simulink model "SmartTraffic"  (R2024b)
settings: Solver=VariableStepAuto  StartTime=0.0  StopTime=10.0  RelTol=1e-3
values from neighbouring files (symbols this model uses):
  dt = 1    [initTraffic.m]
  L_road = 5    [initTraffic.m]
  serviceRate = 2    [genTrafficData.m]    (also in initTraffic.m = 1)
libraries: fuzblock x1
settings Model: Creator=AJCaps  LastModifiedBy=AJCaps

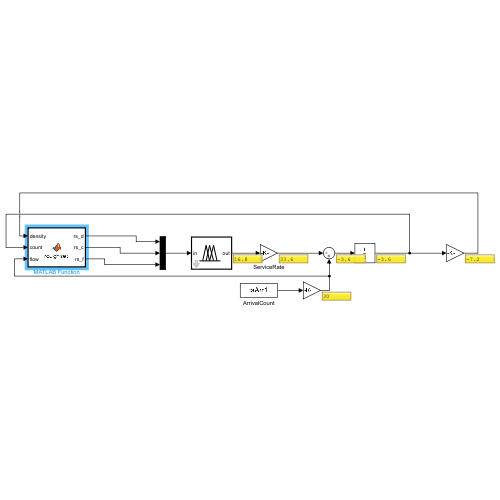
[thumbnail: Simulink's stored preview of the top-level diagram]
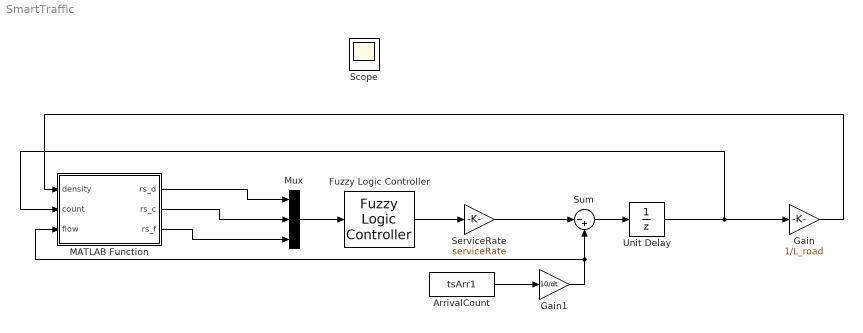
== system SmartTraffic ==
  ArrivalCount : FromWorkspace  VariableName=tsArr1
  Fuzzy Logic Controller : fuzblock/Fuzzy Logic  Controller  FIS='traffic_controller'  OutputSampleNumber=101  DataType=double  FuzzifiedInputs=off  RuleFiringStrengths=off  RuleOutputs=off  AggregatedOutputs=off  SimulateUsing=Interpreted execution  OutOfRangeInputValueMessage=warning  NoRuleFiredMessage=warning  EmptyOutputFuzzySetMessage=warning
  Gain : Gain  Gain=1/L_road
  Gain1 : Gain  Gain=10/dt
  MATLAB Function : MATLAB Function  TreatAsAtomicUnit=on
  Mux : Mux  Inputs=3
  ServiceRate : Gain  Gain=serviceRate
  Sum : Sum  Inputs=|-+
  Unit Delay : UnitDelay  SampleTime=-1  HasFrameUpgradeWarning=on
  Scope : Scope
  wires:
  Gain/1 -> MATLAB Function/1(density)
  Gain1/1 -> Sum/2, MATLAB Function/3(flow)
  MATLAB Function/1(rs_d) -> Mux/1
  Mux/1 -> Fuzzy Logic Controller/1
  Fuzzy Logic Controller/1 -> ServiceRate/1
  ArrivalCount/1 -> Gain1/1
  ServiceRate/1 -> Sum/1
  Sum/1 -> Unit Delay/1
  Unit Delay/1 -> MATLAB Function/2(count), Gain/1
  MATLAB Function/2(rs_c) -> Mux/2
  MATLAB Function/3(rs_f) -> Mux/3

== matlab function SmartTraffic/MATLAB Function ==
  data: density input; rs_d output int8 size=1; count input; flow input; rs_c output int8 size=1; rs_f output int8 size=1
function [rs_d, rs_c, rs_f] = roughset(density, count, flow)
%#codegen
% Density discretization
if density <= 0.2
  rs_d = int8(1);
elseif density <= 0.5
  rs_d = int8(2);
elseif density <= 0.8
  rs_d = int8(3);
else
  rs_d = int8(4);
end

% Count discretization
if count <= 10
  rs_c = int8(1);
elseif count <= 20
  rs_c = int8(2);
elseif count <= 30
  rs_c = int8(3);
else
  rs_c = int8(4);
end

% Flow discretization
if flow <= 100
  rs_f = int8(1);
elseif flow <= 200
  rs_f = int8(2);
elseif flow <= 300
  rs_f = int8(3);
else
  rs_f = int8(4);
end
end
